simulink model "VTOL_CONTROL"  (R2025b)
settings: Solver=VariableStepAuto  StartTime=0.0  StopTime=100  RelTol=1e-3
model workspace (MAT data in the model file):
  M = 1
undefined symbols (not defined in the file): magnitude
settings Model: Creator=Admin  LastModifiedBy=Admin

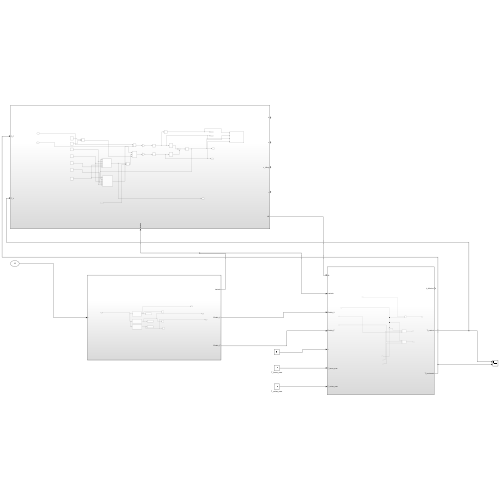
[thumbnail: Simulink's stored preview of the top-level diagram]
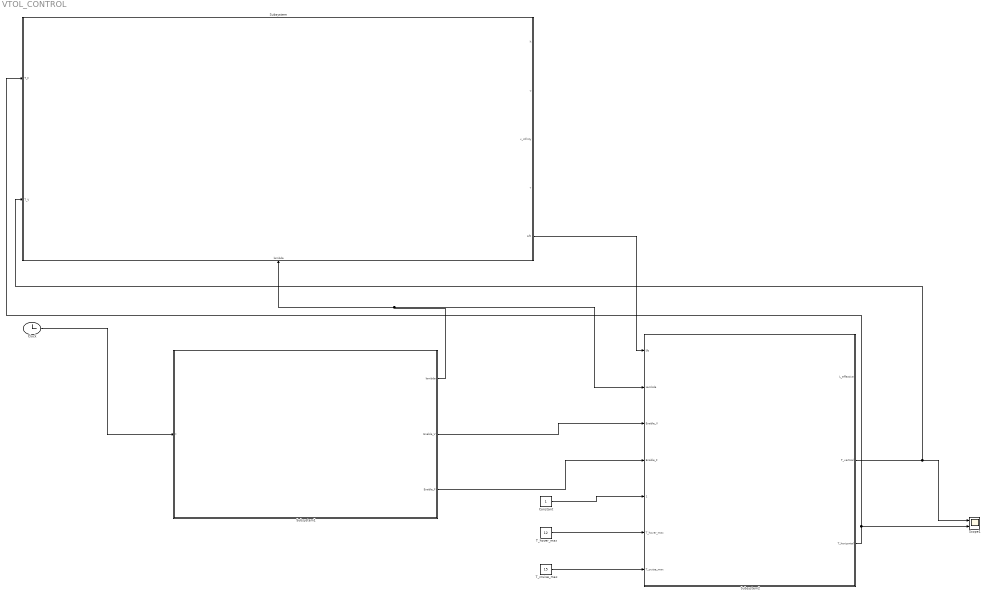
== system VTOL_CONTROL ==
  Clock : Clock
      settings: Decimation=100
  Constant : Constant
  Scope1 : Scope  NumInputPorts=2
      settings: ActiveDisplayYMinimum=-8.2413402976344265  ActiveDisplayYMaximum=30.413621566706912  DataLoggingVariableName=ScopeData4
  Subsystem : Subsystem
      settings: PortSchema="{\"entries\":[{\"content\":{\"sides\":[{\"content\":{\"connectorIds\":[\"In1\",\"In2\"]},\"type\":\"ConnectorPlacement.EquallySpacedRectSide\",\"uuid\":\"717a2cf3-1c0a-44a3-a2ba-538b072e1925\"},{\"content\":{\"connectorIds\":[\"Out1\",\"Out2\",\"Out3\",\"Out4\",\"Out5\"],\"side\":\"RIGHT\"},\"type\":\"ConnectorPlacement.EquallySpacedRectSide\",\"uuid\":\"4d25b5c0-f552-4ea0-9a18-e627fc8b4c8d\"},{\"content\":{\"side\":\"TOP\"},\"type\":\"ConnectorPlacement.EquallySpacedRectSide\",\"uuid\":\"5e6d914d-af3e-475b-a39c-cb9752cea2cc\"},{\"content\":{\"connectorIds\":[\"In3\"],\"side\":\"BOTTOM\"},\"type\":\"ConnectorPlacement.EquallySpacedRectSide\",\"uuid\":\"37b414cc-fcce-4794-8705-d953038efecc\"}]},\"type\":\"ConnectorPlacement.EquallySpacedConnector\",\"uuid\":\"6ac88909-4469-4441-8145-ec1acf4a18cc\"}],\"packageUris\":[\"http://schema.mathworks.com/mf0/Connector/R2020b\"],\"version\":\"1.0\"}"
  Subsystem1 : Subsystem
  Subsystem2 : Subsystem
  T_cruise_max : Constant  Value=15
  T_hover_max : Constant  Value=12
  wires:
  Clock/1 -> Subsystem1/1(t)
  Subsystem1/1(lambda) -> Subsystem2/2(Lambda), Subsystem/3(lambda)
  Subsystem2/3(T_horizontal) -> Subsystem/1(T_F), Scope1/2
  Subsystem2/2(T_vertical) -> Scope1/1, Subsystem/2(T_V)
  Subsystem/5(Lift) -> Subsystem2/1(lift)
  Subsystem1/2(Enable_V) -> Subsystem2/3(Enable_V)
  Subsystem1/3(Enable_F) -> Subsystem2/4(Enable_F)
  Constant/1 -> Subsystem2/5(1)
  T_hover_max/1 -> Subsystem2/6(T_hover_max)
  T_cruise_max/1 -> Subsystem2/7(T_cruise_max)

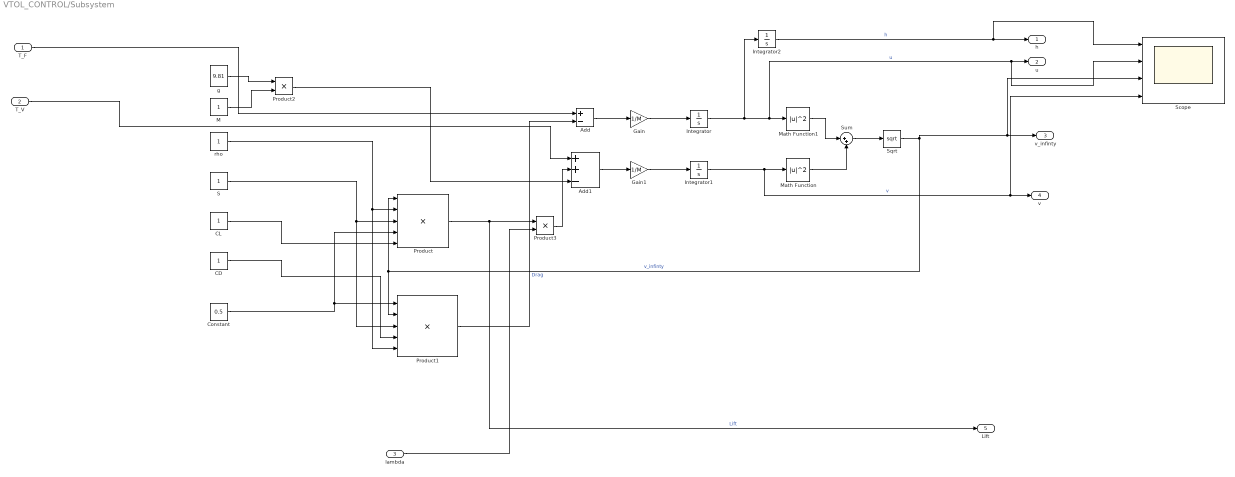
== system VTOL_CONTROL/Subsystem ==
  T_F : Inport
  T_V : Inport  Port=2
  lambda : Inport  Port=3
  Add : Sum  Inputs=+-
  Add1 : Sum  Inputs=++-
  CD : Constant
  CL : Constant
  Constant : Constant  Value=0.5
  Gain : Gain  Gain=1/M
  Gain1 : Gain  Gain=1/M
  Integrator : Integrator
  Integrator1 : Integrator
  Integrator2 : Integrator
  M : Constant
  Math Function : Math  Operator=magnitude^2
  Math Function1 : Math  Operator=magnitude^2
  Product : Product  Inputs=5
  Product1 : Product  Inputs=5
  Product2 : Product
  Product3 : Product
  S : Constant
  Scope : Scope  NumInputPorts=4
      settings: ActiveDisplayYMinimum=-3.9451311540416933E+23  ActiveDisplayYMaximum=6.3219949867021629E+23  DataLoggingVariableName=ScopeData3
  Sqrt : Sqrt
  Sum : Sum  Inputs=|++
  g : Constant  Value=9.81
  rho : Constant
  h : Outport
  u : Outport  Port=2
  v_infinty : Outport  Port=3
  v : Outport  Port=4
  Lift : Outport  Port=5
  wires:
  Integrator/1 -> Integrator2/1, Scope/2, u/1, Math Function1/1  "u"
  Gain/1 -> Integrator/1
  Add/1 -> Gain/1
  rho/1 -> Product1/5, Product/2
  Add1/1 -> Gain1/1
  S/1 -> Product1/3, Product/3
  Constant/1 -> Product/4, Product1/1
  Product1/1 -> Add/2  "Drag"
  Sqrt/1 -> Product/1, Product1/2, Scope/3, v_infinty/1  "v_infinty"
  CD/1 -> Product1/4
  Integrator1/1 -> Scope/4, v/1, Math Function/1  "v"
  Product/1 -> Lift/1, Product3/1  "Lift"
  g/1 -> Product2/1
  CL/1 -> Product/5
  Product2/1 -> Add1/3
  Math Function1/1 -> Sum/1
  Math Function/1 -> Sum/2
  M/1 -> Product2/2
  Gain1/1 -> Integrator1/1
  Sum/1 -> Sqrt/1
  T_F/1 -> Add/1
  T_V/1 -> Add1/1
  Integrator2/1 -> Scope/1, h/1  "h"
  Product3/1 -> Add1/2
  lambda/1 -> Product3/2

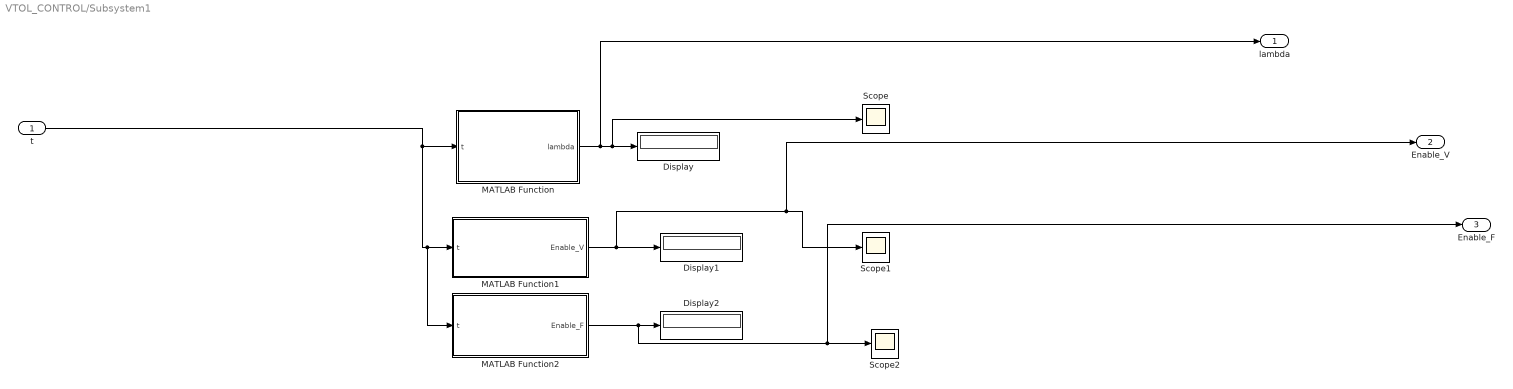
== system VTOL_CONTROL/Subsystem1 ==
  t : Inport
  Display : Display
  Display1 : Display
  Display2 : Display
  MATLAB Function : MATLAB Function  TreatAsAtomicUnit=on
  MATLAB Function1 : MATLAB Function  TreatAsAtomicUnit=on
  MATLAB Function2 : MATLAB Function  TreatAsAtomicUnit=on
  Scope : Scope
      settings: ActiveDisplayYMinimum=-6.6254437632073957  ActiveDisplayYMaximum=9.6738901025392323
  Scope1 : Scope
      settings: ActiveDisplayYMinimum=-0.35557693733498685  ActiveDisplayYMaximum=1.5835833326381588
  Scope2 : Scope
      settings: ActiveDisplayYMinimum=-1.979172228109352  ActiveDisplayYMaximum=3.6933771392759018  DataLoggingVariableName=ScopeData2
  lambda : Outport
  Enable_V : Outport  Port=2
  Enable_F : Outport  Port=3
  wires:
  MATLAB Function2/1(Enable_F) -> Enable_F/1, Scope2/1, Display2/1
  MATLAB Function/1(lambda) -> lambda/1, Scope/1, Display/1
  t/1 -> MATLAB Function2/1(t), MATLAB Function1/1(t), MATLAB Function/1(t)
  MATLAB Function1/1(Enable_V) -> Enable_V/1, Scope1/1, Display1/1

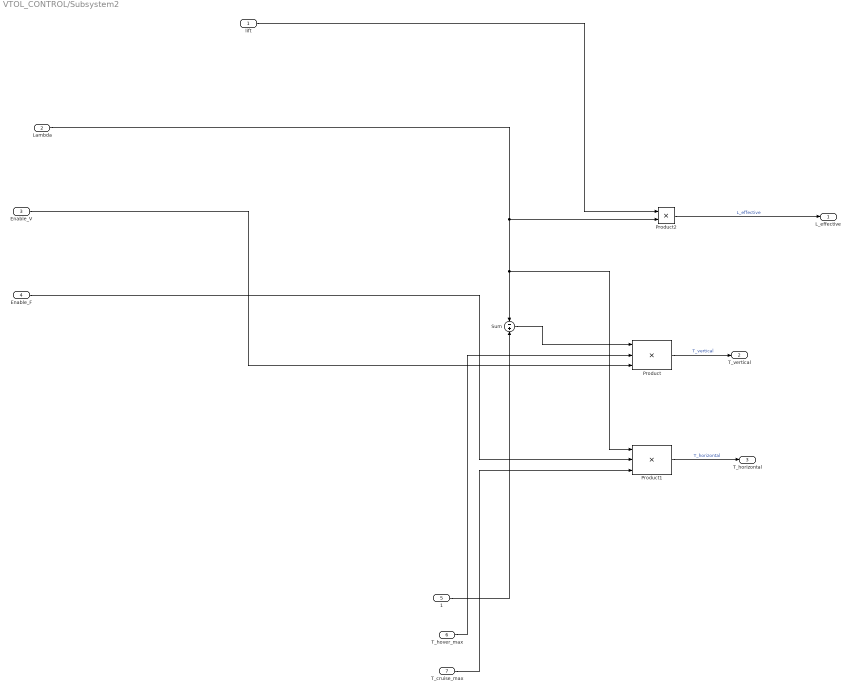
== system VTOL_CONTROL/Subsystem2 ==
  lift : Inport
  Lambda : Inport  Port=2
  Enable_V : Inport  Port=3
  Enable_F : Inport  Port=4
  1 : Inport  Port=5
  T_hover_max : Inport  Port=6
  T_cruise_max : Inport  Port=7
  Product : Product  Inputs=3
  Product1 : Product  Inputs=3
  Product2 : Product
  Sum : Sum  Inputs=-+
  L_effective : Outport
  T_vertical : Outport  Port=2
  T_horizontal : Outport  Port=3
  wires:
  T_hover_max/1 -> Product/2
  Sum/1 -> Product/1
  Lambda/1 -> Product2/2, Product1/1, Sum/1
  Enable_F/1 -> Product1/2
  Product/1 -> T_vertical/1  "T_vertical"
  Product1/1 -> T_horizontal/1  "T_horizontal"
  lift/1 -> Product2/1
  Enable_V/1 -> Product/3
  1/1 -> Sum/2
  Product2/1 -> L_effective/1  "L_effective"
  T_cruise_max/1 -> Product1/3

== matlab function VTOL_CONTROL/Subsystem1/MATLAB Function ==
  data: lambda output; t input
function lambda = blend_factor(t)

if t < 10
    lambda = 0;

elseif t < 30
    a = (t - 10)/20;      % normalized time 0→1
    lambda = a^2;        % parabolic ramp up

elseif t < 65
    lambda = 1;

else
    a = (t - 65)/35;     % normalized time 0→1
    lambda = 1 - a^2;   % parabolic ramp down
end

== matlab function VTOL_CONTROL/Subsystem1/MATLAB Function2 ==
  data: t input; Enable_F output
function Enable_F = enable_forward(t)

% Forward thrust enable logic

if t > 10 && t < 55
    Enable_F = true;     % Transition + Cruise
else
    Enable_F = false;    % Hover, Glide, Back transition
end

== matlab function VTOL_CONTROL/Subsystem1/MATLAB Function1 ==
  data: t input; Enable_V output
function Enable_V = enable_vertical(t)

% Vertical thrust enable logic

if t < 55
    Enable_V = true;     % Hover + Transition + Cruise entry
elseif t >= 65
    Enable_V = true;     % Back transition
else
    Enable_V = false;    % Glide phase (55–65 s)
end
